simulink model "ejercicio1_precompens"  (Simulink 5.0)
settings: Solver=ode45  StartTime=0.0  StopTime=40  RelTol=1e-3
libraries: simulink_extras x1
settings Model: LastModifiedBy=-

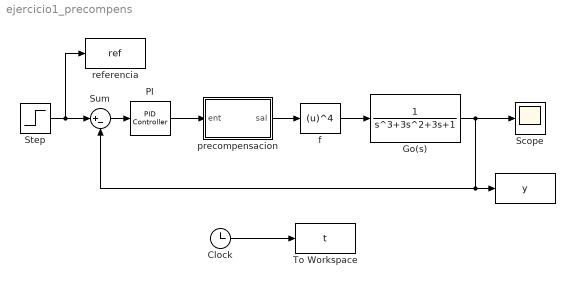
== system ejercicio1_precompens ==
  " " : ToWorkspace  VariableName=y  SampleTime=-1  SaveFormat=Structure
      settings: Decimation=10
  Clock : Clock
      settings: Decimation=10
  Go(s) : TransferFcn  Denominator=[1 3 3 1]
  "PI " : simulink_extras/Additional Linear/PID Controller  P=0.15  I=0.15  D=0
  Scope : Scope
  Step : Step  Time=0  After=0.3  SampleTime=0
  Sum : Sum  Inputs=|+-  SaturateOnIntegerOverflow=on
  To Workspace : ToWorkspace  VariableName=t  SampleTime=-1  SaveFormat=Structure
      settings: Decimation=10
  f : Fcn  Expr=(u)^4
  precompensacion : Subsystem
  "referencia " : ToWorkspace  VariableName=ref  SampleTime=-1  SaveFormat=Structure
      settings: Decimation=10
  wires:
  Step/1 -> Sum/1, "referencia "/1
  Go(s)/1 -> Scope/1, Sum/2, " "/1
  f/1 -> Go(s)/1
  Sum/1 -> "PI "/1
  Clock/1 -> To Workspace/1
  precompensacion/1("sal ") -> f/1
  "PI "/1 -> precompensacion/1(ent)

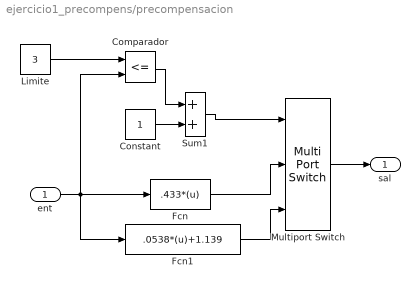
== system ejercicio1_precompens/precompensacion ==
  ent : Inport
  Comparador : RelationalOperator  Operator=<=
  Constant : Constant
  Fcn : Fcn  Expr=.433*(u)
  Fcn1 : Fcn  Expr=.0538*(u)+1.139
  "Limite " : Constant  Value=3
  Multiport Switch : MultiPortSwitch  Inputs=2  SaturateOnIntegerOverflow=on
  Sum1 : Sum  SaturateOnIntegerOverflow=on
  "sal " : Outport
  wires:
  Comparador/1 -> Sum1/1
  Sum1/1 -> Multiport Switch/1
  Multiport Switch/1 -> "sal "/1
  Fcn/1 -> Multiport Switch/2
  Fcn1/1 -> Multiport Switch/3
  "Limite "/1 -> Comparador/1
  ent/1 -> Fcn1/1, Fcn/1, Comparador/2
  Constant/1 -> Sum1/2
